simulink model "ABS_ONOFF_Controller"  (R2014a)
settings: Solver=ode45  SolverMode=SingleTasking  StartTime=0  StopTime=9  FixedStep=0.001  RelTol=1e-3  AbsTol=1e-6
libraries: Solver_SF x1
settings Model: ExtModeTrigMode=oneshot  ExtModeArmWhenConnect=off  Creator=jhu  LastModifiedBy=AUS
settings DataIOCC: LimitDataPoints=off  SignalLoggingSaveFormat=ModelDataLogs  SignalLoggingName=sigsOut
settings OptimizationCC: BlockReduction=off  BooleanDataType=off
settings DebuggingCC: SaveWithParameterizedLinksMsg=none  UnderspecifiedInitializationDetection=Classic  SignalResolutionControl=TryResolveAllWithWarning  SolverPrmCheckMsg=none  MultiTaskDSMMsg=warning  MultiTaskCondExecSysMsg=none  FcnCallInpInsideContextMsg=EnableAllAsWarning  StateNameClashWarn=warning
settings HardwareCC: TargetUnknown=on
settings RTWCC: TemplateMakefile=grt_vc.tmf  IncludeERTFirstTime=on
settings GRTTargetCC: TargetFcnLib=ansi_tfl_tmw.mat  CombineOutputUpdateFcns=off  GRTInterface=on

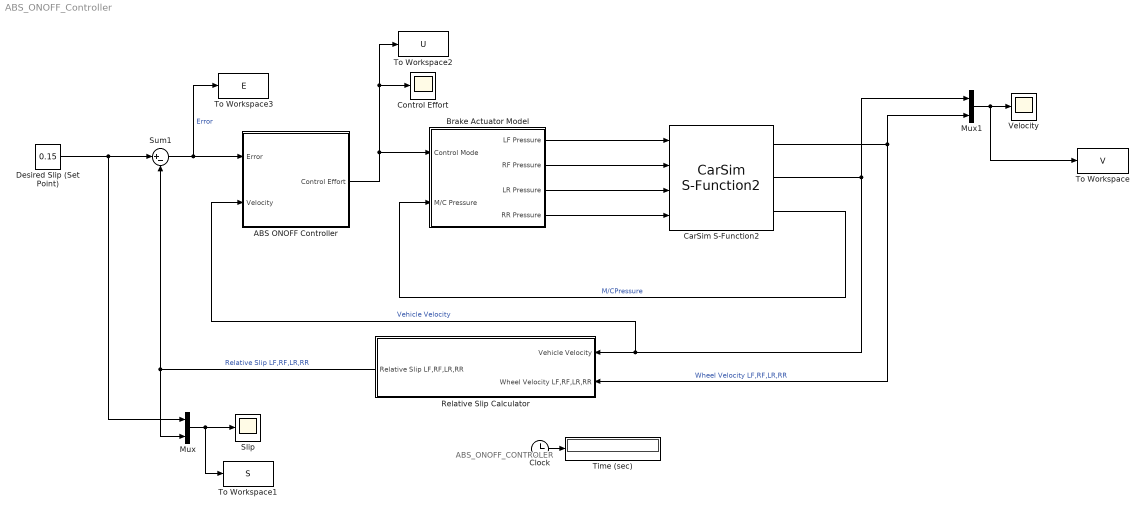
== system ABS_ONOFF_Controller ==
  note: ABS_ONOFF_CONTROLER
  ABS ONOFF Controller : Subsystem
  Brake Actuator Model : Subsystem
  CarSim S-Function2 : Solver_SF/CarSim S-Function2  Priority=1  VehicleCode=i_i  SIMFILE=simfile.sim
      settings: AttributesFormatString=Vehicle Code: %<VehicleCode>
  Clock : Clock
  Control Effort : Scope
      settings: ShowLegends=on  TimeRange=7  YMin=0  YMax=1  SaveName=ScopeData3  MaxDataPoints=50000
  "Desired Slip (Set Point) " : Constant  Value=0.15
  Mux : Mux  Inputs=2
  Mux1 : Mux  Inputs=2
  Relative Slip Calculator : Subsystem
  Slip : Scope
      settings: ShowLegends=on  TimeRange=7  YMin=0  YMax=1  MaxDataPoints=50000
  Sum1 : Sum  Inputs=|+-
  Time (sec) : Display
      settings: Format=bank  Decimation=100
  To Workspace : ToWorkspace  VariableName=V  SaveFormat=Timeseries  SampleTime=0.002
  To Workspace1 : ToWorkspace  VariableName=S  SaveFormat=Timeseries  SampleTime=0.002
  To Workspace2 : ToWorkspace  VariableName=U  SaveFormat=Timeseries  SampleTime=0.002
  To Workspace3 : ToWorkspace  VariableName=E  SaveFormat=Timeseries  SampleTime=0.002
  Velocity : Scope
      settings: ShowLegends=on  YMax=65  MaxDataPoints=50000
  wires:
  CarSim S-Function2/2 -> ABS ONOFF Controller/2(Velocity), Relative Slip Calculator/1(Vehicle Velocity), Mux1/1  "Vehicle Velocity"
  CarSim S-Function2/1 -> Relative Slip Calculator/2(Wheel Velocity LF,RF,LR,RR), Mux1/2  "Wheel Velocity LF,RF,LR,RR"
  Clock/1 -> Time (sec)/1
  Mux/1 -> To Workspace1/1, Slip/1
  Relative Slip Calculator/1(Relative Slip LF,RF,LR,RR) -> Sum1/2, Mux/2  "Relative Slip LF,RF,LR,RR"
  Sum1/1 -> To Workspace3/1, ABS ONOFF Controller/1(Error)  "Error"
  "Desired Slip (Set Point) "/1 -> Mux/1, Sum1/1
  ABS ONOFF Controller/1(Control Effort) -> Brake Actuator Model/1(Control Mode), To Workspace2/1, Control Effort/1
  CarSim S-Function2/3 -> Brake Actuator Model/2(M/C Pressure)  "M/CPressure"
  Brake Actuator Model/1(LF Pressure) -> CarSim S-Function2/1
  Brake Actuator Model/2(RF Pressure) -> CarSim S-Function2/2
  Brake Actuator Model/3(LR Pressure) -> CarSim S-Function2/3
  Brake Actuator Model/4(RR Pressure) -> CarSim S-Function2/4
  Mux1/1 -> To Workspace/1, Velocity/1

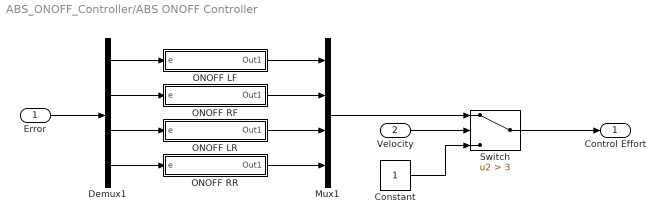
== system ABS_ONOFF_Controller/ABS ONOFF Controller ==
  Error : Inport
  Velocity : Inport  Port=2
  Constant : Constant
  Demux1 : Demux
  Mux1 : Mux
  ONOFF LF : Subsystem
  ONOFF LR : Subsystem
  ONOFF RF : Subsystem
  ONOFF RR : Subsystem
  Switch : Switch  Criteria=u2 > Threshold  Threshold=3
  Control Effort : Outport
  wires:
  Velocity/1 -> Switch/2
  Constant/1 -> Switch/3
  Mux1/1 -> Switch/1
  Switch/1 -> Control Effort/1
  Error/1 -> Demux1/1
  Demux1/1 -> ONOFF LF/1(e)
  ONOFF LF/1(Out1) -> Mux1/1
  Demux1/2 -> ONOFF RF/1(e)
  ONOFF RF/1(Out1) -> Mux1/2
  Demux1/3 -> ONOFF LR/1(e)
  ONOFF LR/1(Out1) -> Mux1/3
  Demux1/4 -> ONOFF RR/1(e)
  ONOFF RR/1(Out1) -> Mux1/4

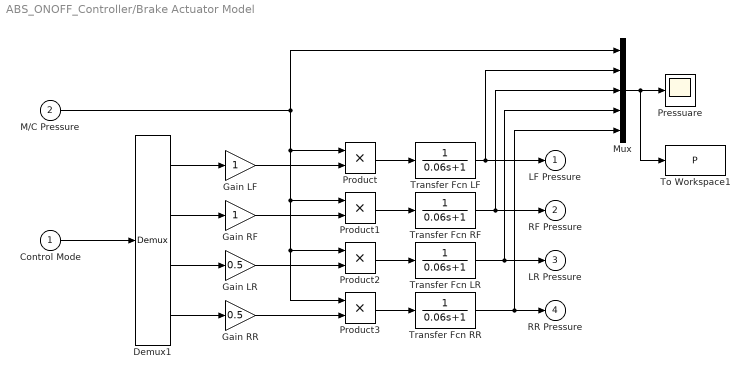
== system ABS_ONOFF_Controller/Brake Actuator Model ==
  Control Mode : Inport
  M/C Pressure : Inport  Port=2
  Demux1 : Demux
  Gain LF : Gain  SaturateOnIntegerOverflow=on  OutDataTypeStr=Inherit: Same as input  ParamDataTypeStr=Inherit: Same as input
  Gain LR : Gain  Gain=0.5  SaturateOnIntegerOverflow=on  OutDataTypeStr=Inherit: Same as input  ParamDataTypeStr=Inherit: Same as input
  Gain RF : Gain  SaturateOnIntegerOverflow=on  OutDataTypeStr=Inherit: Same as input  ParamDataTypeStr=Inherit: Same as input
  Gain RR : Gain  Gain=0.5  SaturateOnIntegerOverflow=on  OutDataTypeStr=Inherit: Same as input  ParamDataTypeStr=Inherit: Same as input
  Mux : Mux  Inputs=5
  Pressuare : Scope
      settings: ShowLegends=on  SaveName=ScopeData9
  Product{,1..3} (4 alike) : Product  SaturateOnIntegerOverflow=on  InputSameDT=on  OutDataTypeStr=Inherit: Same as first input
  To Workspace1 : ToWorkspace  VariableName=P  SaveFormat=Timeseries  SampleTime=0.002
  Transfer Fcn LF : TransferFcn  Denominator=[0.06 1]
  Transfer Fcn LR : TransferFcn  Denominator=[0.06 1]
  Transfer Fcn RF : TransferFcn  Denominator=[0.06 1]
  Transfer Fcn RR : TransferFcn  Denominator=[0.06 1]
  LF Pressure : Outport  InitialOutput=0
  RF Pressure : Outport  Port=2  InitialOutput=0
  LR Pressure : Outport  Port=3  InitialOutput=0
  RR Pressure : Outport  Port=4  InitialOutput=0
  wires:
  Control Mode/1 -> Demux1/1
  Gain LF/1 -> Product/2
  Gain RF/1 -> Product1/2
  Gain LR/1 -> Product2/2
  Gain RR/1 -> Product3/2
  M/C Pressure/1 -> Product/1, Product1/1, Product2/1, Product3/1, Mux/1
  Product/1 -> Transfer Fcn LF/1
  Product1/1 -> Transfer Fcn RF/1
  Product2/1 -> Transfer Fcn LR/1
  Product3/1 -> Transfer Fcn RR/1
  Demux1/1 -> Gain LF/1
  Demux1/2 -> Gain RF/1
  Demux1/3 -> Gain LR/1
  Demux1/4 -> Gain RR/1
  Transfer Fcn LF/1 -> Mux/2, LF Pressure/1
  Transfer Fcn RF/1 -> Mux/3, RF Pressure/1
  Transfer Fcn LR/1 -> Mux/4, LR Pressure/1
  Mux/1 -> To Workspace1/1, Pressuare/1
  Transfer Fcn RR/1 -> Mux/5, RR Pressure/1

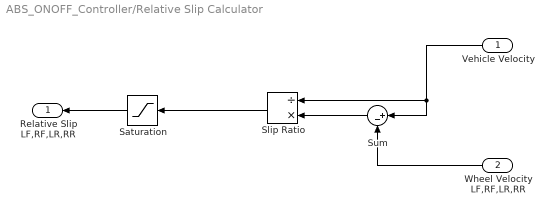
== system ABS_ONOFF_Controller/Relative Slip Calculator ==
  Vehicle Velocity : Inport
  Wheel Velocity LF,RF,LR,RR : Inport  Port=2
  Saturation : Saturate  UpperLimit=1  LowerLimit=0
  Slip Ratio : Product  Inputs=/*  SaturateOnIntegerOverflow=on  InputSameDT=on  OutDataTypeStr=Inherit: Same as first input
  Sum : Sum  Inputs=|+-
  Relative Slip LF,RF,LR,RR : Outport
  wires:
  Vehicle Velocity/1 -> Slip Ratio/1, Sum/1
  Wheel Velocity LF,RF,LR,RR/1 -> Sum/2
  Sum/1 -> Slip Ratio/2
  Slip Ratio/1 -> Saturation/1
  Saturation/1 -> Relative Slip LF,RF,LR,RR/1

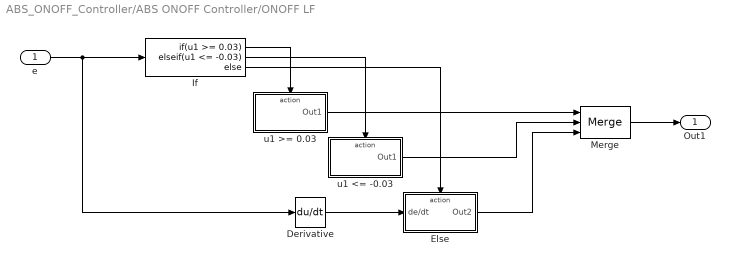
== system ABS_ONOFF_Controller/ABS ONOFF Controller/ONOFF LF ==
  e : Inport
  Derivative : Derivative
  Else : Subsystem  TreatAsAtomicUnit=on
  If : If  IfExpression=u1 >= 0.03  ElseIfExpressions=u1 <= -0.03
  Merge : Merge  Inputs=3
  "u1 <= -0.03 " : Subsystem  TreatAsAtomicUnit=on
  "u1 >= 0.03 " : Subsystem  TreatAsAtomicUnit=on
  Out1 : Outport
  wires:
  "u1 <= -0.03 "/1(Out1) -> Merge/2
  "u1 >= 0.03 "/1(Out1) -> Merge/1
  e/1 -> Derivative/1, If/1
  If/1 -> "u1 >= 0.03 "/Action
  If/2 -> "u1 <= -0.03 "/Action
  Merge/1 -> Out1/1
  If/3 -> Else/Action
  Else/1(Out2) -> Merge/3
  Derivative/1 -> Else/1(de/dt)

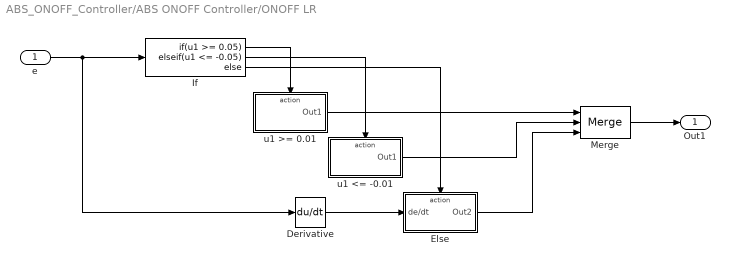
== system ABS_ONOFF_Controller/ABS ONOFF Controller/ONOFF LR ==
  e : Inport
  Derivative : Derivative
  Else : Subsystem  TreatAsAtomicUnit=on
  If : If  IfExpression=u1 >= 0.05  ElseIfExpressions=u1 <= -0.05
  Merge : Merge  Inputs=3
  u1 <= -0.01 : Subsystem  TreatAsAtomicUnit=on
  u1 >= 0.01 : Subsystem  TreatAsAtomicUnit=on
  Out1 : Outport
  wires:
  u1 <= -0.01/1(Out1) -> Merge/2
  u1 >= 0.01/1(Out1) -> Merge/1
  e/1 -> Derivative/1, If/1
  If/1 -> u1 >= 0.01/Action
  If/2 -> u1 <= -0.01/Action
  Merge/1 -> Out1/1
  If/3 -> Else/Action
  Else/1(Out2) -> Merge/3
  Derivative/1 -> Else/1(de/dt)

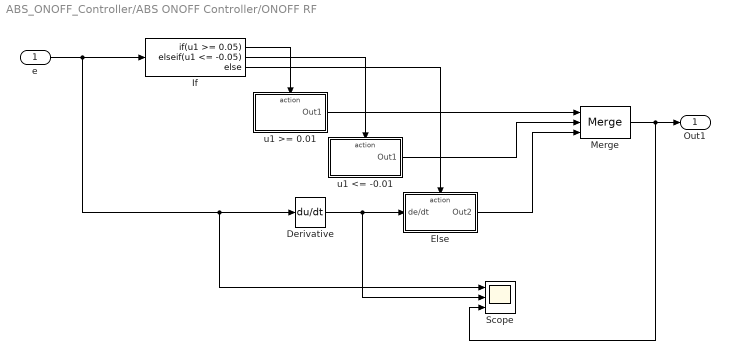
== system ABS_ONOFF_Controller/ABS ONOFF Controller/ONOFF RF ==
  e : Inport
  Derivative : Derivative
  Else : Subsystem  TreatAsAtomicUnit=on
  If : If  IfExpression=u1 >= 0.05  ElseIfExpressions=u1 <= -0.05
  Merge : Merge  Inputs=3
  Scope : Scope  NumInputPorts=3
      settings: YMin=-0.15~-0.012~1  YMax=0.2~0.005~1  SaveName=ScopeData2
  u1 <= -0.01 : Subsystem  TreatAsAtomicUnit=on
  u1 >= 0.01 : Subsystem  TreatAsAtomicUnit=on
  Out1 : Outport
  wires:
  u1 <= -0.01/1(Out1) -> Merge/2
  u1 >= 0.01/1(Out1) -> Merge/1
  e/1 -> Scope/1, Derivative/1, If/1
  If/1 -> u1 >= 0.01/Action
  If/2 -> u1 <= -0.01/Action
  Merge/1 -> Scope/3, Out1/1
  If/3 -> Else/Action
  Else/1(Out2) -> Merge/3
  Derivative/1 -> Scope/2, Else/1(de/dt)

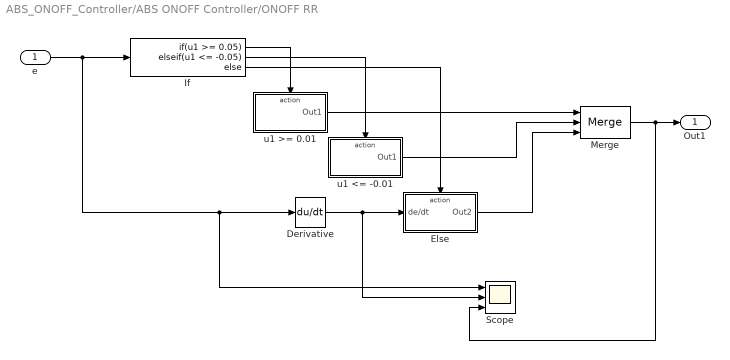
== system ABS_ONOFF_Controller/ABS ONOFF Controller/ONOFF RR ==
  e : Inport
  Derivative : Derivative
  Else : Subsystem  TreatAsAtomicUnit=on
  If : If  IfExpression=u1 >= 0.05  ElseIfExpressions=u1 <= -0.05
  Merge : Merge  Inputs=3
  Scope : Scope  NumInputPorts=3
      settings: YMin=-0.15~-0.012~0.95  YMax=0.2~0.005~1.05  SaveName=ScopeData2
  u1 <= -0.01 : Subsystem  TreatAsAtomicUnit=on
  u1 >= 0.01 : Subsystem  TreatAsAtomicUnit=on
  Out1 : Outport
  wires:
  u1 <= -0.01/1(Out1) -> Merge/2
  u1 >= 0.01/1(Out1) -> Merge/1
  e/1 -> Scope/1, Derivative/1, If/1
  If/1 -> u1 >= 0.01/Action
  If/2 -> u1 <= -0.01/Action
  Merge/1 -> Scope/3, Out1/1
  If/3 -> Else/Action
  Else/1(Out2) -> Merge/3
  Derivative/1 -> Scope/2, Else/1(de/dt)

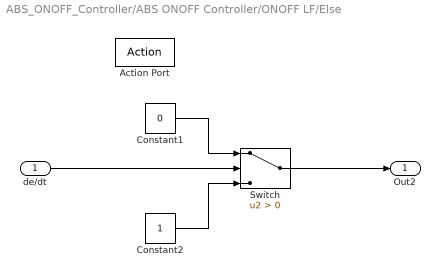
== system ABS_ONOFF_Controller/ABS ONOFF Controller/ONOFF LF/Else ==
  de/dt : Inport
  Action Port : ActionPort  ActionType=else
  Constant1 : Constant  Value=0
  Constant2 : Constant
  Switch : Switch  Criteria=u2 > Threshold
  Out2 : Outport
  wires:
  de/dt/1 -> Switch/2
  Switch/1 -> Out2/1
  Constant2/1 -> Switch/3
  Constant1/1 -> Switch/1

== system ABS_ONOFF_Controller/ABS ONOFF Controller/ONOFF LF/u1 <= -0.03  ==
  Action Port : ActionPort  ActionType=elseif
  Constant : Constant  Value=0
  Out1 : Outport
  wires:
  Constant/1 -> Out1/1

== system ABS_ONOFF_Controller/ABS ONOFF Controller/ONOFF LF/u1 >= 0.03  ==
  Action Port : ActionPort  ActionType=then
  Constant : Constant
  Out1 : Outport
  wires:
  Constant/1 -> Out1/1

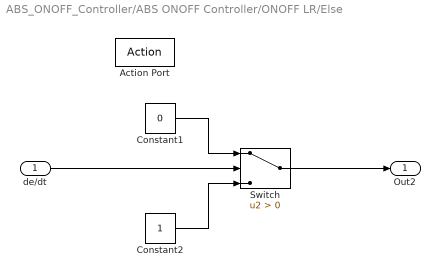
== system ABS_ONOFF_Controller/ABS ONOFF Controller/ONOFF LR/Else ==
  de/dt : Inport
  Action Port : ActionPort  ActionType=else
  Constant1 : Constant  Value=0
  Constant2 : Constant
  Switch : Switch  Criteria=u2 > Threshold
  Out2 : Outport
  wires:
  de/dt/1 -> Switch/2
  Switch/1 -> Out2/1
  Constant2/1 -> Switch/3
  Constant1/1 -> Switch/1

== system ABS_ONOFF_Controller/ABS ONOFF Controller/ONOFF LR/u1 <= -0.01 ==
  Action Port : ActionPort  ActionType=elseif
  Constant : Constant  Value=0
  Out1 : Outport
  wires:
  Constant/1 -> Out1/1

== system ABS_ONOFF_Controller/ABS ONOFF Controller/ONOFF LR/u1 >= 0.01 ==
  Action Port : ActionPort  ActionType=then
  Constant : Constant
  Out1 : Outport
  wires:
  Constant/1 -> Out1/1

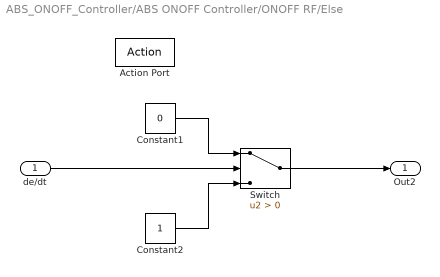
== system ABS_ONOFF_Controller/ABS ONOFF Controller/ONOFF RF/Else ==
  de/dt : Inport
  Action Port : ActionPort  ActionType=else
  Constant1 : Constant  Value=0
  Constant2 : Constant
  Switch : Switch  Criteria=u2 > Threshold
  Out2 : Outport
  wires:
  de/dt/1 -> Switch/2
  Switch/1 -> Out2/1
  Constant2/1 -> Switch/3
  Constant1/1 -> Switch/1

== system ABS_ONOFF_Controller/ABS ONOFF Controller/ONOFF RF/u1 <= -0.01 ==
  Action Port : ActionPort  ActionType=elseif
  Constant : Constant  Value=0
  Out1 : Outport
  wires:
  Constant/1 -> Out1/1

== system ABS_ONOFF_Controller/ABS ONOFF Controller/ONOFF RF/u1 >= 0.01 ==
  Action Port : ActionPort  ActionType=then
  Constant : Constant
  Out1 : Outport
  wires:
  Constant/1 -> Out1/1

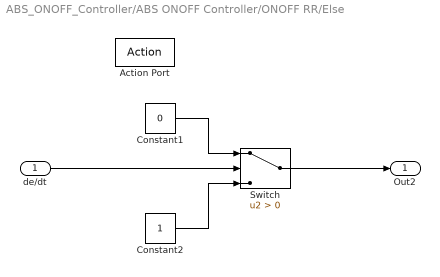
== system ABS_ONOFF_Controller/ABS ONOFF Controller/ONOFF RR/Else ==
  de/dt : Inport
  Action Port : ActionPort  ActionType=else
  Constant1 : Constant  Value=0
  Constant2 : Constant
  Switch : Switch  Criteria=u2 > Threshold
  Out2 : Outport
  wires:
  de/dt/1 -> Switch/2
  Switch/1 -> Out2/1
  Constant2/1 -> Switch/3
  Constant1/1 -> Switch/1

== system ABS_ONOFF_Controller/ABS ONOFF Controller/ONOFF RR/u1 <= -0.01 ==
  Action Port : ActionPort  ActionType=elseif
  Constant : Constant  Value=0
  Out1 : Outport
  wires:
  Constant/1 -> Out1/1

== system ABS_ONOFF_Controller/ABS ONOFF Controller/ONOFF RR/u1 >= 0.01 ==
  Action Port : ActionPort  ActionType=then
  Constant : Constant
  Out1 : Outport
  wires:
  Constant/1 -> Out1/1
